simulink model "final_SM"  (R2024b)
settings: Solver=VariableStepAuto  StartTime=0.0  StopTime=10.0  RelTol=1e-3
settings Model: Creator=gobin  LastModifiedBy=gobin

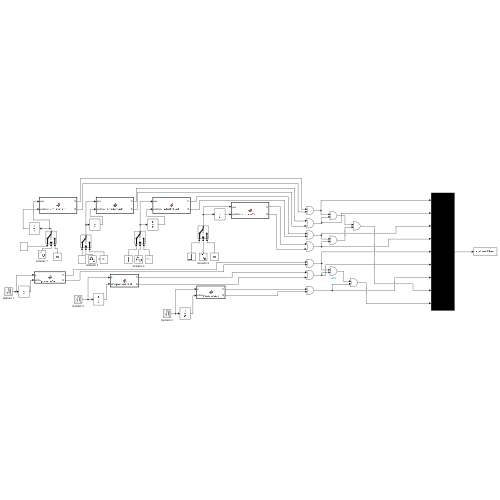
[thumbnail: Simulink's stored preview of the top-level diagram]
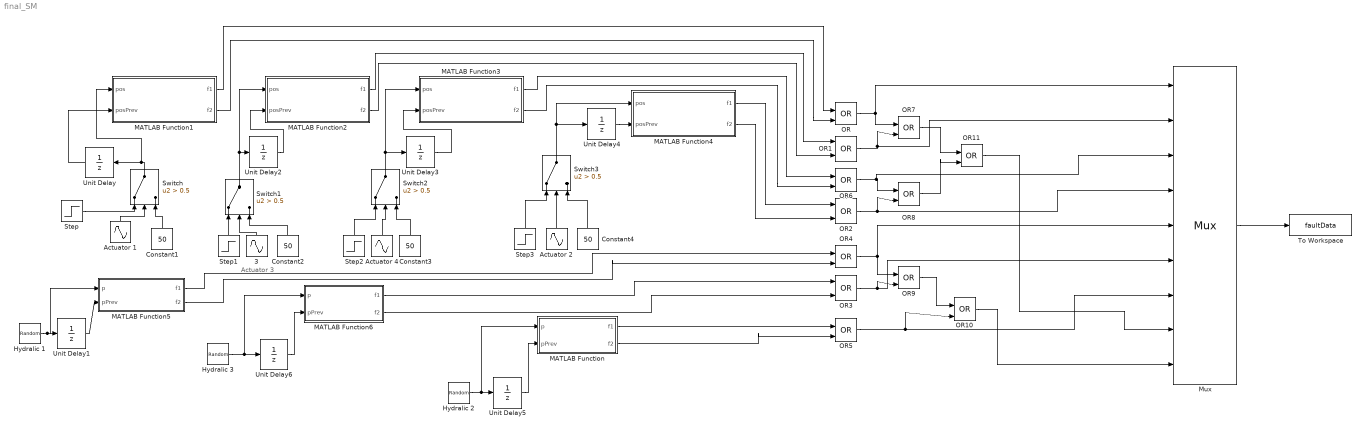
== system final_SM ==
  note: Actuator 3
  " 3" : Sin  Amplitude=5  SampleTime=0.01
  Actuator 1 : Sin  Amplitude=5  SampleTime=0.01
  Actuator 2 : Sin  Amplitude=5  SampleTime=0.01
  Actuator 4 : Sin  Amplitude=5  SampleTime=0.01
  Constant{1..4} (4 alike) : Constant  Value=50
  Hydralic 1 : RandomNumber  Mean=1250  Variance=150^2  SampleTime=0.01
  Hydralic 2 : RandomNumber  Mean=1250  Variance=150^2  SampleTime=0.01
  Hydralic 3 : RandomNumber  Mean=1250  Variance=150^2  SampleTime=0.01
  MATLAB Function : MATLAB Function  TreatAsAtomicUnit=on
  MATLAB Function1 : MATLAB Function  TreatAsAtomicUnit=on
  MATLAB Function2 : MATLAB Function  TreatAsAtomicUnit=on
  MATLAB Function3 : MATLAB Function  TreatAsAtomicUnit=on
  MATLAB Function4 : MATLAB Function  TreatAsAtomicUnit=on
  MATLAB Function5 : MATLAB Function  TreatAsAtomicUnit=on
  MATLAB Function6 : MATLAB Function  TreatAsAtomicUnit=on
  Mux : Mux  Inputs=9
  OR{,1..11} (12 alike) : Logic  Operator=OR  IconShape=distinctive  AllPortsSameDT=off  OutDataTypeStr=boolean
  Step{,1..3} (4 alike) : Step  Time=2  SampleTime=0
  Switch{,1..3} (4 alike) : Switch  Criteria=u2 > Threshold  Threshold=0.5  SaturateOnIntegerOverflow=off  InputSameDT=off
  To Workspace : ToWorkspace  VariableName=faultData  SampleTime=-1
  Unit Delay{,1..6} (7 alike) : UnitDelay  SampleTime=0.01  HasFrameUpgradeWarning=on
  wires:
  Unit Delay/1 -> MATLAB Function1/2(posPrev)
  Unit Delay2/1 -> MATLAB Function2/2(posPrev)
  Unit Delay3/1 -> MATLAB Function3/2(posPrev)
  Unit Delay4/1 -> MATLAB Function4/2(posPrev)
  Hydralic 1/1 -> MATLAB Function5/1(p), Unit Delay1/1
  Unit Delay1/1 -> MATLAB Function5/2(pPrev)
  Unit Delay6/1 -> MATLAB Function6/2(pPrev)
  Hydralic 3/1 -> Unit Delay6/1, MATLAB Function6/1(p)
  Unit Delay5/1 -> MATLAB Function/2(pPrev)
  Hydralic 2/1 -> Unit Delay5/1, MATLAB Function/1(p)
  MATLAB Function1/1(f1) -> OR/1
  MATLAB Function1/2(f2) -> OR/2
  MATLAB Function2/1(f1) -> OR1/1
  MATLAB Function2/2(f2) -> OR1/2
  MATLAB Function3/1(f1) -> OR6/1
  MATLAB Function3/2(f2) -> OR6/2
  MATLAB Function4/1(f1) -> OR2/1
  MATLAB Function4/2(f2) -> OR2/2
  MATLAB Function5/1(f1) -> OR4/1
  MATLAB Function5/2(f2) -> OR4/2
  MATLAB Function6/1(f1) -> OR3/1
  MATLAB Function6/2(f2) -> OR3/2
  MATLAB Function/1(f1) -> OR5/1
  MATLAB Function/2(f2) -> OR5/2
  Mux/1 -> To Workspace/1
  Actuator 1/1 -> Switch/2
  Switch/1 -> MATLAB Function1/1(pos), Unit Delay/1
  Step/1 -> Switch/1
  Constant1/1 -> Switch/3
  Switch1/1 -> Unit Delay2/1, MATLAB Function2/1(pos)
  Step1/1 -> Switch1/1
  " 3"/1 -> Switch1/2
  Constant2/1 -> Switch1/3
  Actuator 4/1 -> Switch2/2
  Constant3/1 -> Switch2/3
  Step2/1 -> Switch2/1
  Switch2/1 -> Unit Delay3/1, MATLAB Function3/1(pos)
  Actuator 2/1 -> Switch3/2
  Constant4/1 -> Switch3/3
  Step3/1 -> Switch3/1
  Switch3/1 -> Unit Delay4/1, MATLAB Function4/1(pos)
  OR1/1 -> Mux/2, OR7/2
  OR6/1 -> Mux/3, OR8/1
  OR2/1 -> Mux/4, OR8/2
  OR4/1 -> Mux/5, OR9/1
  OR3/1 -> Mux/6, OR9/2
  OR5/1 -> Mux/7, OR10/2
  OR9/1 -> OR10/1
  OR8/1 -> OR11/2
  OR7/1 -> OR11/1
  OR/1 -> Mux/1, OR7/1
  OR11/1 -> Mux/8
  OR10/1 -> Mux/9

== matlab function final_SM/MATLAB Function2 ==
  data: pos input; f1 output; posPrev input; f2 output
function [f1, f2] = actuatorFault(pos, posPrev)
f1 = abs(pos) > 10;                % Out of bounds
f2 = abs(pos - posPrev) > 5;      % Rapid movement
end

== matlab function final_SM/MATLAB Function3 ==
  data: pos input; f1 output; posPrev input; f2 output
function [f1, f2] = actuatorFault(pos, posPrev)
f1 = abs(pos) > 10;                % Out of bounds
f2 = abs(pos - posPrev) > 5;      % Rapid movement
end

== matlab function final_SM/MATLAB Function4 ==
  data: pos input; f1 output; posPrev input; f2 output
function [f1, f2] = actuatorFault(pos, posPrev)
f1 = abs(pos) > 10;                % Out of bounds
f2 = abs(pos - posPrev) > 5;      % Rapid movement
end

== matlab function final_SM/MATLAB Function ==
  data: p input; f1 output; pPrev input; f2 output
function [f1, f2] = pressureFault(p, pPrev)
f1 = (p < 500) | (p > 1500);      % Out of range
f2 = abs(p - pPrev) > 100;         % Rapid change
end

== matlab function final_SM/MATLAB Function5 ==
  data: p input; f1 output; pPrev input; f2 output
function [f1, f2] = pressureFault(p, pPrev)
f1 = (p < 500) | (p > 1500);      % Out of range
f2 = abs(p - pPrev) > 100;         % Rapid change
end

== matlab function final_SM/MATLAB Function6 ==
  data: p input; f1 output; pPrev input; f2 output
function [f1, f2] = pressureFault(p, pPrev)
f1 = (p < 500) | (p > 1500);      % Out of range
f2 = abs(p - pPrev) > 100;         % Rapid change
end

== matlab function final_SM/MATLAB Function1 ==
  data: pos input; f1 output; posPrev input; f2 output
function [f1, f2] = actuatorFault(pos, posPrev)
f1 = abs(pos) > 10;                % Out of bounds
f2 = abs(pos - posPrev) > 4;      % Rapid movement
end
